simulink model "dummy_plot"  (R2024b)
settings: Solver=VariableStepAuto  StartTime=0.0  StopTime=100  MaxStep=0.001  RelTol=1e-3
undefined symbols (not defined in the file): d, D, omega_M, P_INIT_EKF, Q_INIT, r, R_5, T_a, T_c, T_s, x_coords, y_coords, Z_INIT_EKF
settings Model: PacingRate=1000  Creator=alber  LastModifiedBy=Enrico
settings DataIOCC: ReturnWorkspaceOutputs=off
settings DebuggingCC: UnderSpecifiedDimensionMsg=warning
settings RTWCC: GPUComputeCapability=3.5

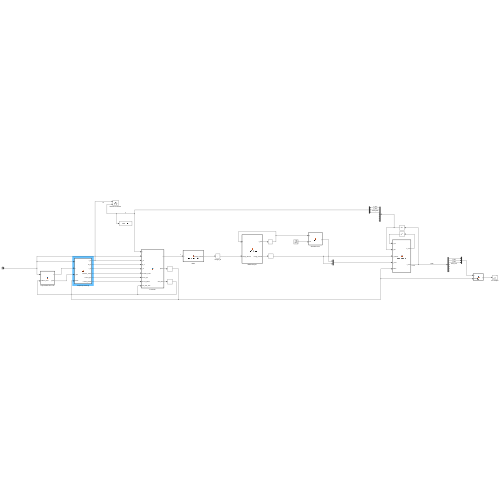
[thumbnail: Simulink's stored preview of the top-level diagram]
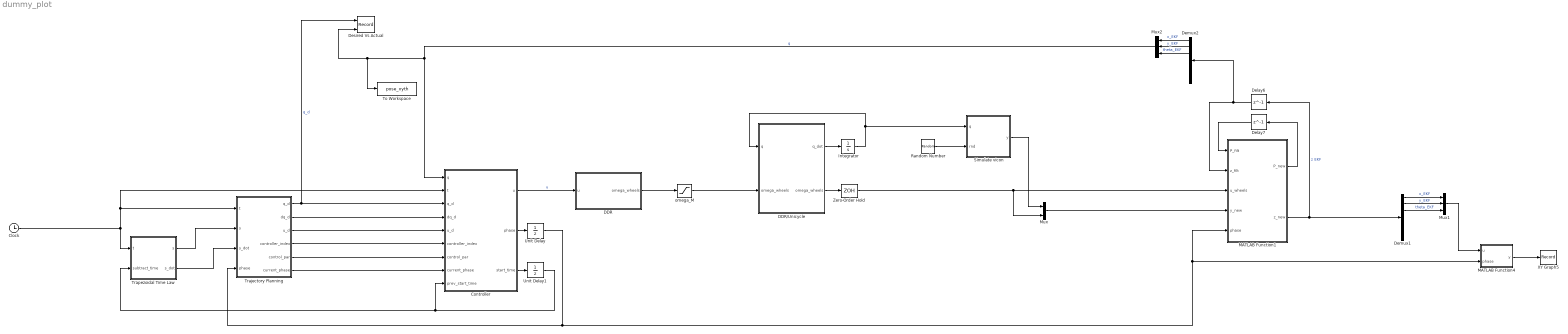
== system dummy_plot ==
  Clock : Clock
  Controller : MATLAB Function  TreatAsAtomicUnit=on
  DDR : MATLAB Function  TreatAsAtomicUnit=on
  DDR/Unicycle : MATLAB Function  TreatAsAtomicUnit=on
  Delay6 : Delay  DelayLength=1  InitialCondition=Z_INIT_EKF  SampleTime=T_s
  Delay7 : Delay  DelayLength=1  InitialCondition=P_INIT_EKF  SampleTime=T_s
  Demux1 : Demux  Outputs=7
  Demux2 : Demux  Outputs=7
  "Desired Vs Actual " : Record  FileSettingsInternal="{\"entries\":[{\"content\":{\"excelSettings\":{\"content\":{},\"type\":\"Streamout.ExcelSettings\"}},\"type\":\"Streamout.FileSettingStorage\",\"uuid\":\"\"}],\"packageUris\":[\"http:\\/\\/schema.mathworks.com\\/mf0\\/streamout_blocks\\/R2020a\"],\"version\":\"1.0\"}"  Layout=[1 1]  SignalsInternal="{\"entries\":[{\"content\":{\"signals\":[{\"content\":{\"blockPath\":[],\"dimensions\":[3,1],\"domain\":\"\",\"hasChildren\":true,\"lineColor\":\"#139fff\",\"lineWidth\":2,\"port\":1,\"sid\":[\"\"],\"signalID\":1,\"signalName\":\"q_d\"},\"type\":\"RecordBlkView.Signal\",\"uuid\":\"\"},{\"content\":{\"blockPath\":[],\"channel\":[1,1],\"dimensions\":[3,1],\"domain\":\"\",\"lineColor\":\"#0072bd\",\"lineWidth\":2,\"parentID\":1,\"plots\":[ 1 ],\"port\":1,\"sid\":[\"\"],\"signalID\":2,\"signalName\":\"q_d\"},\"type\":\"RecordBlkView.Signal\",\"uuid\":\"\"},{\"content\":{\"blockPath\":[],\"dimensions\":[3],\"domain\":\"\",\"hasChildren\":true,\"lineColor\":\"#b746ff\",\"lineWidth\":2,\"port\":2,\"sid\":[\"\"],\"signalID\":3,\"signalName\":\"q\"},\"type\":\"RecordBlkView.Signal\",\"uuid\":\"\"},{\"content\":{\"blockPath\":[],\"channel\":[1],\"dimensions\":[3],\"domain\":\"\",\"lineColor\":\"#edb120\",\"lineWidth\":2,\"parentID\":3,\"plots\":[ 1 ],\"port\":2,\"sid\":[\"\"],\"signalID\":4,\"signalName\":\"q\"},\"type\":\"RecordBlkView.Signal\",\"uuid\":\"\"},{\"content\":{\"blockPath\":[],\"channel\":[2,1],\"dimensions\":[3,1],\"domain\":\"\",\"lineColor\":\"#d95319\",\"lineWidth\":2,\"parentID\":1,\"plots\":[ 1 ],\"port\":1,\"sid\":[\"\"],\"signalID\":5,\"signalName\":\"q_d\"},\"type\":\"RecordBlkView.Signal\",\"uuid\":\"\"},{\"content\":{\"blockPath\":[],\"channel\":[3,1],\"dimensions\":[3,1],\"domain\":\"\",\"lineColor\":\"#edb120\",\"lineWidth\":2,\"parentID\":1,\"port\":1,\"sid\":[\"\"],\"signalID\":6,\"signalName\":\"q_d\"},\"type\":\"RecordBlkView.Signal\",\"uuid\":\"\"},{\"content\":{\"blockPath\":[],\"channel\":[2],\"dimensions\":[3],\"domain\":\"\",\"lineColor\":\"#139fff\",\"lineWidth\":2,\"parentID\":3,\"plots\":[ 1 ],\"port\":2,\"sid\":[\"\"],\"signalID\":7,\"signalName\":\"q\"},\"type\":\"RecordBlkView.Signal\",\"uuid\":\"\"},{\"content\":{\"blockPath\":[],\"channel\":[3],\"dimensions\":[3],\"domain\":\"\",\"lineColor\":\"#ff6929\",\"lineWidth\":2,\"parentID\":3,\"port\":2,\"sid\":[\"\"],\"signalID\":8,\"signalName\":\"q\"},\"type\":\"RecordBlkView.Signal\",\"uuid\":\"\"}]},\"type\":\"RecordBlkView.InputSignals\",\"uuid\":\"\"}],\"packageUris\":[\"http:\\/\\/schema.mathworks.com\\/mf0\\/streamout_blocks\\/R2020a\"],\"version\":\"1.0\"}"  VisualizationBindings="{\"xyplotplugin\":{\"info\":[{\"series\":[{\"bindingParametersList\":[{\"parameter\":\"X-Axis\",\"signalID\":4,\"signalName\":\"q(1)\"},{\"parameter\":\"Y-Axis\",\"signalID\":7,\"signalName\":\"q(2)\"}],\"seriesID\":0},{\"bindingParametersList\":[{\"parameter\":\"X-Axis\",\"signalID\":2,\"signalName\":\"q_d(1,1)\"},{\"parameter\":\"Y-Axis\",\"signalID\":5,\"signalName\":\"q_d(2,1)\"}],\"seriesID\":1}],\"subplotID\":1}]}}"  CompatibilityTag=XY
  Integrator : Integrator  InitialCondition=Q_INIT
  MATLAB Function1 : MATLAB Function  TreatAsAtomicUnit=on
  MATLAB Function4 : MATLAB Function  TreatAsAtomicUnit=on
  Mux : Mux  Inputs=2
  Mux1 : Mux  Inputs=3
  Mux2 : Mux  Inputs=3
  Random Number : RandomNumber  SampleTime=0.1
  Simulate vicon : MATLAB Function  TreatAsAtomicUnit=on
  To Workspace : ToWorkspace  VariableName=pose_xyth  SampleTime=-1
  Trajectory Planning : MATLAB Function  TreatAsAtomicUnit=on
  Trapezoidal Time Law : MATLAB Function  TreatAsAtomicUnit=on
  Unit Delay : UnitDelay  InitialCondition=1  SampleTime=T_s  HasFrameUpgradeWarning=on
  Unit Delay1 : UnitDelay  InitialCondition=inf  SampleTime=T_s  HasFrameUpgradeWarning=on
  XY Graph5 : Record  FileSettingsInternal="{\"entries\":[{\"content\":{\"excelSettings\":{\"content\":{},\"type\":\"Streamout.ExcelSettings\"}},\"type\":\"Streamout.FileSettingStorage\",\"uuid\":\"\"}],\"packageUris\":[\"http:\\/\\/schema.mathworks.com\\/mf0\\/streamout_blocks\\/R2020a\"],\"version\":\"1.0\"}"  Layout=[1 1]  SignalsInternal="{\"entries\":[{\"content\":{\"signals\":[{\"content\":{\"blockPath\":[],\"dimensions\":[3,1],\"domain\":\"\",\"hasChildren\":true,\"lineColor\":\"#22b573\",\"lineWidth\":2,\"port\":1,\"sid\":[\"\"],\"signalID\":1,\"signalName\":\"MATLAB Function4\"},\"type\":\"RecordBlkView.Signal\",\"uuid\":\"\"},{\"content\":{\"blockPath\":[],\"channel\":[1,1],\"dimensions\":[3,1],\"domain\":\"\",\"lineColor\":\"#0072bd\",\"lineWidth\":2,\"parentID\":1,\"plots\":[ 1 ],\"port\":1,\"sid\":[\"\"],\"signalID\":2,\"signalName\":\"MATLAB Function4\"},\"type\":\"RecordBlkView.Signal\",\"uuid\":\"\"},{\"content\":{\"blockPath\":[],\"channel\":[2,1],\"dimensions\":[3,1],\"domain\":\"\",\"lineColor\":\"#4dbeee\",\"lineWidth\":2,\"parentID\":1,\"plots\":[ 1 ],\"port\":1,\"sid\":[\"\"],\"signalID\":3,\"signalName\":\"MATLAB Function4\"},\"type\":\"RecordBlkView.Signal\",\"uuid\":\"\"},{\"content\":{\"blockPath\":[],\"channel\":[3,1],\"dimensions\":[3,1],\"domain\":\"\",\"lineColor\":\"#a2142f\",\"lineWidth\":2,\"parentID\":1,\"port\":1,\"sid\":[\"\"],\"signalID\":4,\"signalName\":\"MATLAB Function4\"},\"type\":\"RecordBlkView.Signal\",\"uuid\":\"\"}]},\"type\":\"RecordBlkView.InputSignals\",\"uuid\":\"\"}],\"packageUris\":[\"http:\\/\\/schema.mathworks.com\\/mf0\\/streamout_blocks\\/R2020a\"],\"version\":\"1.0\"}"  VisualizationBindings="{\"xyplotplugin\":{\"info\":[{\"series\":[{\"bindingParametersList\":[{\"parameter\":\"X-Axis\",\"signalID\":2,\"signalName\":\"MATLAB Function4(1,1)\"},{\"parameter\":\"Y-Axis\",\"signalID\":3,\"signalName\":\"MATLAB Function4(2,1)\"}],\"seriesID\":0}],\"subplotID\":1}]}}"  CompatibilityTag=XY
  Zero-Order Hold : ZeroOrderHold  SampleTime=T_s
  omega_M : Saturate  UpperLimit=omega_M  LowerLimit=-omega_M
  wires:
  Trajectory Planning/1(q_d) -> "Desired Vs Actual "/1, Controller/3(q_d)  "q_d"
  Trajectory Planning/2(dq_d) -> Controller/4(dq_d)
  Trajectory Planning/3(u_d) -> Controller/5(u_d)
  Trajectory Planning/4(controller_index) -> Controller/6(controller_index)
  Trajectory Planning/5(control_par) -> Controller/7(control_par)
  MATLAB Function1/2(z_new) -> Demux1/1, Delay6/1  "z EKF"
  Delay7/1 -> MATLAB Function1/1(P_filt)
  Demux1/2 -> Mux1/2  "y_EKF"
  MATLAB Function1/1(P_new) -> Delay7/1
  Demux1/3 -> Mux1/3  "theta_EKF"
  Demux1/1 -> Mux1/1  "x_EKF"
  DDR/1(omega_wheels) -> omega_M/1
  Controller/1(u) -> DDR/1(u)  "u"
  Mux/1 -> MATLAB Function1/4(y_new)
  Clock/1 -> Controller/2(t), Trajectory Planning/1(t), Trapezoidal Time Law/1(t)
  Unit Delay/1 -> Trajectory Planning/4(phase), MATLAB Function4/2(phase), MATLAB Function1/5(phase)
  Trapezoidal Time Law/1(s) -> Trajectory Planning/2(s)
  Random Number/1 -> Simulate vicon/2(rnd)
  Simulate vicon/1(y) -> Mux/1
  Integrator/1 -> DDR/Unicycle/1(q), Simulate vicon/1(q)
  Trajectory Planning/6(current_phase) -> Controller/8(current_phase)
  Controller/3(start_time) -> Unit Delay1/1
  Unit Delay1/1 -> Trapezoidal Time Law/2(subtract_time), Controller/9(prev_start_time)
  Zero-Order Hold/1 -> MATLAB Function1/3(u_wheels), Mux/2
  Trapezoidal Time Law/2(s_dot) -> Trajectory Planning/3(s_dot)
  DDR/Unicycle/1(q_dot) -> Integrator/1
  omega_M/1 -> DDR/Unicycle/2("omega_wheels ")
  DDR/Unicycle/2(omega_wheels) -> Zero-Order Hold/1
  Controller/2(phase) -> Unit Delay/1
  Mux1/1 -> MATLAB Function4/1(u)
  MATLAB Function4/1(y) -> XY Graph5/1
  Mux2/1 -> To Workspace/1, "Desired Vs Actual "/2, Controller/1(q)  "q"
  Delay6/1 -> MATLAB Function1/2(z_filt), Demux2/1
  Demux2/2 -> Mux2/2  "y_EKF"
  Demux2/3 -> Mux2/3  "theta_EKF"
  Demux2/1 -> Mux2/1  "x_EKF"

== matlab function dummy_plot/DDR ==
  data: u input; omega_wheels output; r parameter; d parameter
function omega_wheels = kin2omegawheels(u, r, d)
omega_l = u(1)/r-d/(2*r)*u(2);
omega_r = u(1)/r+d/(2*r)*u(2);
omega_wheels = [omega_l;omega_r];

== matlab function dummy_plot/DDR//Unicycle ==
  data: q input; omega_wheels input; q_dot output; omega_wheels output; d parameter; r parameter
function [q_dot,  omega_wheels]  = DDR_Unicycle(q, omega_wheels, d, r)
omega_wheels = omega_wheels;
u = [r*(omega_wheels(1)+omega_wheels(2))/2; r*(-omega_wheels(1)+omega_wheels(2))/d];

q_dot = [cos(q(3))*u(1);
    sin(q(3))*u(1);
    u(2)];

end

== matlab function dummy_plot/MATLAB Function4 ==
  data: u input; y output; phase input
function y = fcn(u, phase)
if phase == 3   
    y = u;
% orange area entrance
else 
    y = [1; -0.3;0];
end

== matlab function dummy_plot/Trapezoidal Time Law ==
  data: s output; t input; T_a parameter; s_dot output; T_c parameter; subtract_time input
function [s,s_dot]=fcn(t, T_a, T_c, subtract_time)

    v_c = 1 / (T_a + T_c);
    a = v_c / T_a;
    
    % we get the start time of the trajectory tracking 
    t = t - subtract_time;

    if(t < 0)
        s_dot = 0;
        s = 0;
    elseif(t > 2*T_a+T_c)
        s_dot = 0;
        s = 1;
    elseif(t > T_a+T_c)
        s_dot = v_c - a * (t - T_a - T_c);
        s = (a * T_a^2)/2 + v_c * (t - T_a - T_c) + v_c * (T_c) - (a * (t - T_c - T_a)^2)/2;
    elseif(t > T_a)
        s_dot = v_c; 
        s = (a * T_a^2)/2 + v_c * (t - T_a);
    else 
        s_dot = a * t;
        s = (a * t^2)/2;
    end
    
end

== matlab function dummy_plot/Simulate vicon ==
  data: q input; rnd input; y output; x_coords parameter; y_coords parameter
function y = fcn(q, rnd, x_coords, y_coords)

if (q(1) > x_coords(5) && q(1) < x_coords(6) && q(2) > y_coords(1) && q(2) < y_coords(5))

    % red area
    y = [0;0;0];

elseif (q(1) > x_coords(7) && q(1) < x_coords(9) && q(2) > y_coords(1) && q(2) < y_coords(6))

    % orange area 
    if(rnd < 0.1)
        y = q;
    else 
        y = [0;0;0];
    end 
    
else 
    
    % white area
    y = q;

end

%bypass
y = q;

== matlab function dummy_plot/Trajectory Planning ==
  data: x_coords parameter; y_coords parameter; t input; s input; s_dot input; phase input; q_d output; dq_d output; u_d output; controller_index output; control_par output; current_phase output
function [q_d,dq_d,u_d,controller_index,control_par,current_phase] = fcn(x_coords,y_coords,t, s, s_dot,phase)

% regulation
if phase == 1

    controller_index = 1;

    q_d = [x_coords(2);y_coords(2);0];
    dq_d = [0;0;0];
    u_d = [0;0];
    control_par = [0.2,0.5,1];
    current_phase = 1;

% Cartesian polinomials
elseif phase == 2   

    controller_index = 2;

    q_i = [x_coords(2), y_coords(2), 0];
    q_f = [x_coords(8), y_coords(4), 0];
    k_i = 6;
    k_f = 6; 
    k_sign = sign(k_i);

    y = [0,0,0,0;0,0,0,0];
    y(1,1) = q_f(1);
    y(1,2) = q_i(1);
    y(1,3) = k_f * cos(q_f(3)) - 3 * q_f(1);
    y(1,4) = k_i * cos(q_i(3)) + 3 * q_i(1);

    y(2,1) = q_f(2);
    y(2,2) = q_i(2);
    y(2,3) = k_f * sin(q_f(3)) - 3 * q_f(2);
    y(2,4) = k_i * sin(q_i(3)) + 3 * q_i(2);
    

    x_exp = y(1,1) * s^3 - y(1,2) * (s - 1)^3 + y(1,3) * s^2 * (s - 1) + y(1,4) * s * (s - 1)^2;
    y_exp = y(2,1) * s^3 - y(2,2) * (s - 1)^3 + y(2,3) * s^2 * (s - 1) + y(2,4) * s * (s - 1)^2;

    x_dot = 3 * y(1,1) * s^2 - 3 * y(1,2) * (s-1)^2 + 2 * y(1,3) * s * (s-1) + y(1,3) * s^2 + y(1,4) * (s-1)^2 + 2 * y(1,4) * s * (s-1);
    y_dot = 3 * y(2,1) * s^2 - 3 * y(2,2) * (s-1)^2 + 2 * y(2,3) * s * (s-1) + y(2,3) * s^2 + y(2,4) * (s-1)^2 + 2 * y(2,4) * s * (s-1);
    x_dotdot = 6 * y(1,1) * s - 6 * y(1,2) * (s-1) + 2 * y(1,3) * s + 2 * y(1,3) * (s-1) + 2 * s * y(1,3) + 2 * y(1,4) * (s-1) + 2 * y(1,4) * s + 2 * y(1,4) * (s-1);
    y_dotdot = 6 * y(2,1) * s - 6 * y(2,2) * (s-1) + 2 * y(2,3) * s + 2 * y(2,3) * (s-1) + 2 * s * y(2,3) + 2 * y(2,4) * (s-1) + 2 * y(2,4) * s + 2 * y(2,4) * (s-1);
    
    
    if(k_sign == 1)
        v = sqrt((x_dot)^2 + (y_dot)^2) * s_dot;
        theta_exp = atan2(y_dot,x_dot) + pi;
    else
        v = - sqrt((x_dot)^2 + (y_dot)^2) * s_dot;
        theta_exp = atan2(y_dot,x_dot);
    end

    q_d = [x_exp; y_exp; wrapToPi(theta_exp)];

    w = (((x_dot) * (y_dotdot) - (y_dot) * (x_dotdot)) / ((x_dot)^2 + (y_dot)^2)) * s_dot;

    u_d = [v;w];

    x_prime = x_dot * s_dot;
    y_prime = y_dot * s_dot;

    dq_d = [x_prime; y_prime; w];

    control_par = [0.1,0.1,0.01];

    current_phase = 2;

% circle and a half
elseif phase == 3

    controller_index = 2;
    R = 0.5;
    T_trj = 40;
    omega = 2 * pi / T_trj;
    % 1.5 turns: multiply omega by 1.5 for theta
    theta = 1.5 * omega * t;
    
    x_d = 1.95 + R * cos(theta);
    dx_d = -R * 1.5 * omega * sin(theta);
    ddx_d = -R * (1.5 * omega)^2 * cos(theta);
    
    y_d = R * sin(theta);
    dy_d = R * 1.5 * omega * cos(theta);
    ddy_d = -R * (1.5 * omega)^2 * sin(theta);
    
    theta_d = atan2(dy_d, dx_d);
    dtheta_d = (dx_d * ddy_d - dy_d * ddx_d) / (dx_d^2 + dy_d^2);
    
    q_d = [x_d; y_d; theta_d];
    dq_d = [dx_d; dy_d; dtheta_d];
    u_d = [sqrt(dx_d^2 + dy_d^2); dtheta_d];
    
    control_par = [0.1, 0.1, 0.01];
    current_phase = 3;
else

    controller_index=1;

    q_d = [x_coords(2);y_coords(2);0];
    dq_d = [0;0;0];
    u_d = [0;0];
    control_par = [0,0,0];

    current_phase = 4;
 

end


end

== matlab function dummy_plot/Controller ==
  data: u output size=[2,1]; q input; t input; q_d input; dq_d input; u_d input; controller_index input; control_par input; x_coords parameter; y_coords parameter; current_phase input; prev_start_time input; phase output size=1; start_time output size=1
function [u,phase,start_time]  = fcn(q, t, q_d, dq_d, u_d, controller_index, control_par, x_coords, y_coords, current_phase,prev_start_time)

if controller_index == 1
    % posture regulation
    % transform q
    % compute pointing error
    phase = 1;
    start_time = prev_start_time;

    R = [cos(q_d(3)), sin(q_d(3)), 0;
        -sin(q_d(3)), cos(q_d(3)), 0;
        0, 0, 1];
    p_prime = R*(q - q_d);
    rho = sqrt(p_prime(1)^2 + p_prime(2)^2);
    gamma = wrapToPi(atan2(p_prime(2), p_prime(1))+pi-p_prime(3));
    delta = p_prime(3) + gamma;
    if abs(gamma)<1e-4
        u = [control_par(1)*rho*cos(gamma); control_par(2)*gamma + control_par(1)*cos(gamma)*(gamma + control_par(3)*delta)];
    else
        u = [control_par(1)*rho*cos(gamma); control_par(2)*gamma + control_par(1)*sin(gamma)*cos(gamma)*(gamma + control_par(3)*delta)/gamma];
    end

    % switch to next phase feedback linearization
    if abs(q(1) - x_coords(2)) <= 0.05 && abs(q(2) - y_coords(2)) <= 0.05
        phase = 2;
        start_time = t;
    end

else %if controller_index == 2

    start_time = prev_start_time;

    % feedback linearization
    p = [q_d(1)+control_par(3)*cos(q_d(3)); q_d(2)+control_par(3)*sin(q_d(3))];
    p_dot = [dq_d(1)-control_par(3)*sin(q_d(3))*dq_d(3); dq_d(2)+control_par(3)*cos(q_d(3))*dq_d(3)];
    e_tilde = p-[q(1)+control_par(3)*cos(q(3)); q(2)+control_par(3)*sin(q(3))];
    k1 = control_par(1);
    k2 = control_par(2);
    K = [k1, 0; 0, k2];
    in = K * e_tilde;
    u = [cos(q(3)), sin(q(3)); -sin(q(3))/control_par(3), cos(q(3))/control_par(3)]*(p_dot+in);

    if  current_phase == 2
        % switch to next phase, circle around obstacle at [1.45; -0.3]
        if abs(q(1) - x_coords(8)) <= 0.1 && abs(q(2) - y_coords(4)) <= 0.1
            phase = 3;
        else
            phase = 2;
        end
    else
        phase = 3;
    end

end

end

== matlab function dummy_plot/MATLAB Function1 ==
  data: P_filt input; P_new output; z_filt input; z_new output; u_wheels input; y_new input; D parameter; R_5 parameter; T_s parameter; r parameter; d parameter; phase input
function [P_new, z_new] = EKF_filtering(P_filt, z_filt, u_wheels, y_new, D, R_5, T_s, r, d, phase)

v_k = r * (z_filt(6) + z_filt(7))/2;
w_k = r * (z_filt(7) - z_filt(6))/d;
theta_mean = z_filt(3) + (w_k * T_s)/2;

F_k = [1, 0, -T_s * v_k * sin(theta_mean), 0, 0, T_s * r * cos(theta_mean)/2 + (T_s)^2 * r * v_k * sin(theta_mean)/(2*d), T_s * r * cos(theta_mean)/2 - (T_s)^2 * r * v_k * sin(theta_mean)/(2*d);
    0, 1, T_s * v_k * cos(theta_mean), 0, 0, T_s * r * sin(theta_mean)/2 - (T_s)^2 * r * v_k * cos(theta_mean)/(2*d), T_s * r * sin(theta_mean)/2 + (T_s)^2 * r * v_k * cos(theta_mean)/(2*d);
    0, 0, 1, 0, 0, (-T_s*r)/d, (T_s*r)/d;
    0, 0, 0, 0, 0, T_s, 0;
    0, 0, 0, 0, 0, 0, T_s;
    0, 0, 0, 0, 0, 0, 0;
    0, 0, 0, 0, 0, 0, 0];

z_pred = [z_filt(1)+(T_s*r*(z_filt(6)+z_filt(7))/2)*cos(theta_mean + (T_s*r*(z_filt(6)+z_filt(7)))/(2*d));
        z_filt(2)+(T_s*r*(z_filt(6)+z_filt(7))/2)*sin(theta_mean + (T_s*r*(z_filt(7)-z_filt(6)))/(2*d));
        theta_mean + (T_s*r*(z_filt(7)-z_filt(6))/(2*d));
        T_s*z_filt(6);
        T_s*z_filt(7);
        u_wheels(1);
        u_wheels(2)];
z_pred(3) = wrapToPi(z_pred(3));

P_pred = F_k * P_filt * F_k' + D;


%% Encoders + GPS
y_new_1 = y_new(1:5);

H = [1, 0, 0, 0, 0, 0, 0;
    0, 1, 0, 0, 0, 0, 0;
    0, 0, 1, 0, 0, 0, 0;
    0, 0, 0, 0, 0, 1, 0;
    0, 0, 0, 0, 0, 0, 1];

e = y_new_1 - H * z_pred;
K = P_pred * H' / (H * P_pred * H' + R_5);

e(3) = wrapToPi(e(3));

z_new = z_pred + K * e;
P_new = P_pred - K * H * P_pred;


end
